simulink model "simpleEqu"  (R2023b)
settings: Solver=VariableStepAuto  StartTime=0.0  StopTime=10.0  RelTol=1e-3
settings Model: Creator=mhagh  LastModifiedBy=mhagh

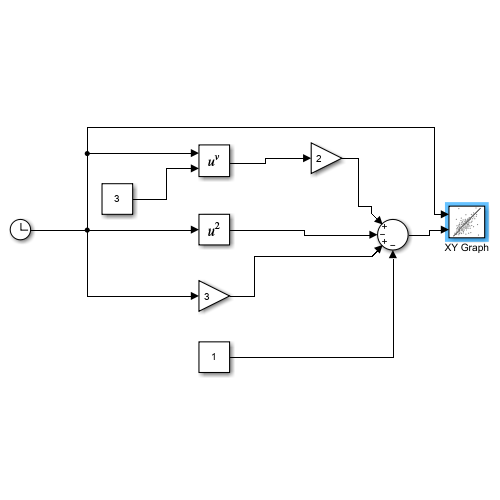
[thumbnail: Simulink's stored preview of the top-level diagram]
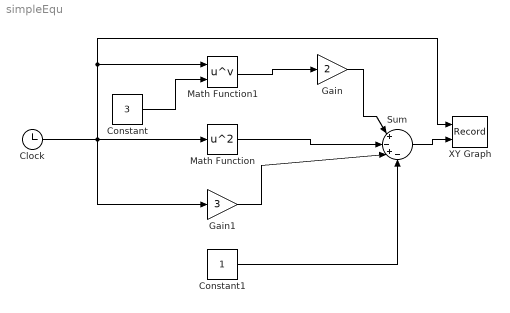
== system simpleEqu ==
  Clock : Clock
  Constant : Constant  Value=3
  Constant1 : Constant
  Gain : Gain  Gain=2
  Gain1 : Gain  Gain=3
  Math Function : Math  Operator=square
  Math Function1 : Math  Operator=pow
  Sum : Sum  Inputs=|+-+-
  XY Graph : Record  FileSettingsInternal="{\"entries\":[{\"content\":{\"excelSettings\":{\"content\":{},\"type\":\"Streamout.ExcelSettings\"}},\"type\":\"Streamout.FileSettingStorage\",\"uuid\":\"\"}],\"packageUris\":[\"http:\\/\\/schema.mathworks.com\\/mf0\\/streamout_blocks\\/R2020a\"],\"version\":\"1.0\"}"  Layout=[1 1]  SignalsInternal="{\"entries\":[{\"content\":{\"signals\":[{\"content\":{\"blockPath\":[],\"dimensions\":[1],\"domain\":\"\",\"lineColor\":\"#a2142f\",\"plots\":[ 1 ],\"port\":1,\"sid\":[\"\"],\"signalID\":1,\"signalName\":\"Clock\"},\"type\":\"RecordBlkView.Signal\",\"uuid\":\"\"},{\"content\":{\"blockPath\":[],\"dimensions\":[1],\"domain\":\"\",\"lineColor\":\"#139fff\",\"plots\":[ 1 ],\"port\":2,\"sid\":[\"\"],\"signalID\":2,\"signalName\":\"Sum\"},\"type\":\"RecordBlkView.Signal\",\"uuid\":\"\"}]},\"type\":\"RecordBlkView.InputSignals\",\"uuid\":\"\"}],\"packageUris\":[\"http:\\/\\/schema.mathworks.com\\/mf0\\/streamout_blocks\\/R2020a\"],\"version\":\"1.0\"}"  VisualizationBindings="{\"xyplotplugin\":{\"info\":[{\"series\":[{\"bindingParametersList\":[{\"parameter\":\"X-Axis\",\"signalID\":1,\"signalName\":\"Clock\"},{\"parameter\":\"Y-Axis\",\"signalID\":2,\"signalName\":\"Sum\"}],\"seriesID\":0}],\"subplotID\":1}]}}"  CompatibilityTag=XY
  wires:
  Constant/1 -> Math Function1/2
  Sum/1 -> XY Graph/2
  Clock/1 -> XY Graph/1, Math Function1/1, Gain1/1, Math Function/1
  Math Function1/1 -> Gain/1
  Gain/1 -> Sum/1
  Math Function/1 -> Sum/2
  Gain1/1 -> Sum/3
  Constant1/1 -> Sum/4
